simulink model "Intake"  (R2021a)
settings: Solver=FixedStepAuto  StartTime=0.0  StopTime=sim_time/4  FixedStep=stepsize  RelTol=1e-3
values from neighbouring files (symbols this model uses):
  AFR = 14.7    [Combustion_Engine.m]    (also in Combustion_Engine_V3.m)
  Bore = 82.7*10^-3    (= 0.0827)    [Combustion_Engine.m]    (also in Combustion_Engine_V3.m)
  Cd = 0.35    [Combustion_Engine.m]    (also in Combustion_Engine_V3.m)
  ConRod = 140*10^-3    (= 0.14)    [Combustion_Engine.m]    (also in Combustion_Engine_V3.m)
  CR = 10    [Combustion_Engine.m]    (also in Combustion_Engine_V3.m)
  CrankRadius = Stroke/2    (= 0.0465)    [Combustion_Engine.m]    (also in Combustion_Engine_V3.m)
  engine_speed = 3000    [Combustion_Engine.m]    (also in Combustion_Engine_V3.m)
  gma = 1.35    [Combustion_Engine.m]    (also in Combustion_Engine_V3.m)
  LHV = 44400*10^3    (= 44400000)    [Combustion_Engine.m]    (also in Combustion_Engine_V3.m)
  m_0 = P_0*(V_comp)/(R*T_air)    (= 5.9876570894e-05)    [Combustion_Engine.m]    (also in Combustion_Engine_V3.m)
  MAP = 80000    [Combustion_Engine.m]    (also in Combustion_Engine_V3.m)
  R = 287    [Combustion_Engine.m]    (also in Combustion_Engine_V3.m)
  Rho = 1.27    [Combustion_Engine.m]    (also in Combustion_Engine_V3.m)
  Stroke = 93*10^-3    (= 0.093)    [Combustion_Engine.m]    (also in Combustion_Engine_V3.m)
  T_air = 323    [Combustion_Engine.m]    (also in Combustion_Engine_V3.m)
  V2 = V_comp    (= 5.55061799844e-05)    [Combustion_Engine.m]    (also in Combustion_Engine_V3.m)
  V_comp = V_cyl/(CR-1)    (= 5.55061799844e-05)    [Combustion_Engine.m]    (also in Combustion_Engine_V3.m)
  V_cyl = (Bore/2)^2*pi*Stroke    (= 0.00049955561986)    [Combustion_Engine.m]    (also in Combustion_Engine_V3.m)
  Valve_dia = 30*10^-3    (= 0.03)    [Combustion_Engine.m]    (also in Combustion_Engine_V3.m)
  Valve_lift = 9*10^-3    (= 0.009)    [Combustion_Engine.m]    (also in Combustion_Engine_V3.m)
settings Model: Creator=rafik  LastModifiedBy=rafik
settings SolverCC: AlgebraicLoopSolver=TrustRegion
settings DataIOCC: ReturnWorkspaceOutputs=off
settings DebuggingCC: MaxConsecutiveZCsMsg=none

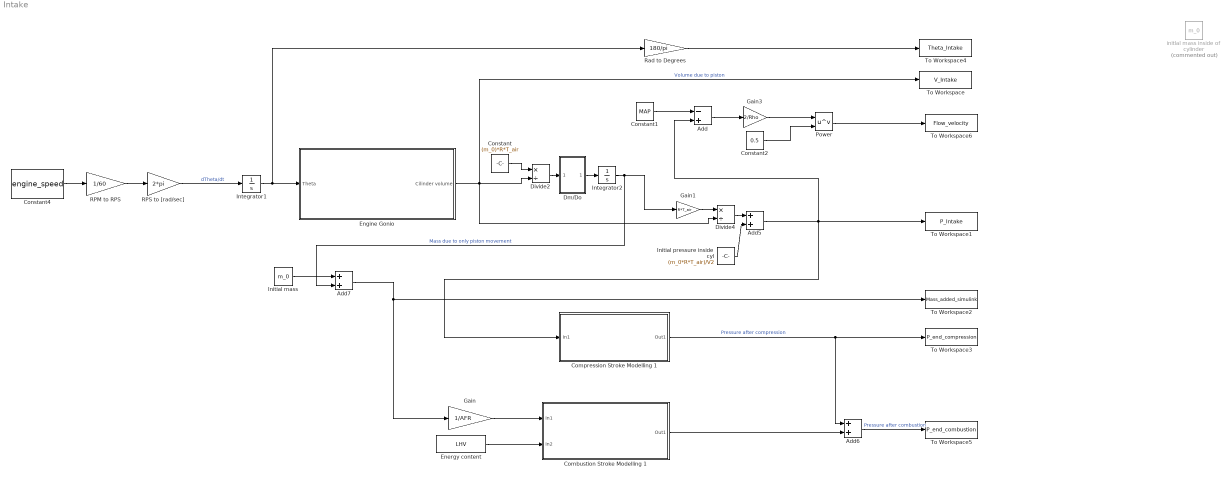
== system Intake ==
  Add : Sum  Inputs=-+
  Add5 : Sum
  Add6 : Sum
  Add7 : Sum
  Combustion Stroke Modelling 1 : Subsystem
  Compression Stroke Modelling 1 : Subsystem
  Constant : Constant  Value=(m_0)*R*T_air
  Constant1 : Constant  Value=MAP
  Constant2 : Constant  Value=0.5
  Constant4 : Constant  Value=engine_speed
  Divide2 : Product  Inputs=*/
  Divide4 : Product  Inputs=*/
  Dm/Do : Subsystem
  Energy content : Constant  Value=LHV
  Engine Gonio : Subsystem
  Gain : Gain  Gain=1/AFR
  Gain1 : Gain  Gain=R*T_air
  Gain3 : Gain  Gain=2/Rho
  "Initial mass " : Constant  Value=m_0
  Initial pressure inside cyl : Constant  Value=(m_0*R*T_air)/V2
  Integrator1 : Integrator  LimitOutput=on  UpperSaturationLimit=pi  LowerSaturationLimit=0
  Integrator2 : Integrator  LimitOutput=on  UpperSaturationLimit=1  LowerSaturationLimit=0
  Power : Math  Operator=pow  SaturateOnIntegerOverflow=on
  "RPM to RPS " : Gain  Gain=1/60
  RPS to [rad/sec] : Gain  Gain=2*pi
  "Rad to Degrees " : Gain  Gain=180/pi
  To Workspace : ToWorkspace  VariableName=V_Intake  SampleTime=-1
  To Workspace1 : ToWorkspace  VariableName=P_Intake  SampleTime=-1
  To Workspace2 : ToWorkspace  VariableName=Mass_added_simulink  SampleTime=-1
  To Workspace3 : ToWorkspace  VariableName=P_end_compression  SampleTime=-1
  To Workspace4 : ToWorkspace  VariableName=Theta_Intake  SampleTime=-1
  To Workspace5 : ToWorkspace  VariableName=P_end_combustion  SampleTime=-1
  To Workspace6 : ToWorkspace  VariableName=Flow_velocity  SampleTime=-1
  initlal mass inside of cylinder : Constant  Commented=on  Value=m_0
  wires:
  Energy content/1 -> Combustion Stroke Modelling 1/2(In2)
  Integrator1/1 -> "Rad to Degrees "/1, Engine Gonio/1(Theta)
  Constant4/1 -> "RPM to RPS "/1
  "RPM to RPS "/1 -> RPS to [rad/sec]/1
  RPS to [rad/sec]/1 -> Integrator1/1  "dTheta/dt"
  Constant/1 -> Divide2/1
  Engine Gonio/1(Cilinder volume) -> To Workspace/1, Divide2/2, Divide4/2  "Volume due to piston"
  Divide2/1 -> Dm/Do/1(In1)
  Gain1/1 -> Divide4/1
  Divide4/1 -> Add5/1
  Add5/1 -> Compression Stroke Modelling 1/1(In1), To Workspace1/1, Add/2
  Initial pressure inside cyl/1 -> Add5/2
  Compression Stroke Modelling 1/1(Out1) -> To Workspace3/1, Add6/1  "Pressure after compression"
  Integrator2/1 -> Add7/2, Gain1/1  "Mass due to only piston movement"
  Combustion Stroke Modelling 1/1(Out1) -> Add6/2
  Add6/1 -> To Workspace5/1  "Pressure after combustion"
  Gain/1 -> Combustion Stroke Modelling 1/1(In1)
  "Initial mass "/1 -> Add7/1
  Add7/1 -> Gain/1, To Workspace2/1
  "Rad to Degrees "/1 -> To Workspace4/1
  Dm/Do/1(Out1) -> Integrator2/1
  Constant1/1 -> Add/1
  Add/1 -> Gain3/1
  Gain3/1 -> Power/1
  Constant2/1 -> Power/2
  Power/1 -> To Workspace6/1

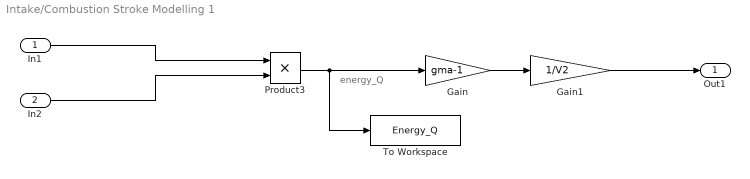
== system Intake/Combustion Stroke Modelling 1 ==
  note: energy_Q
  In1 : Inport
  In2 : Inport  Port=2
  Gain : Gain  Gain=gma-1
  Gain1 : Gain  Gain=1/V2
  Product3 : Product
  To Workspace : ToWorkspace  VariableName=Energy_Q  SaveFormat=Timeseries  SampleTime=-1
  Out1 : Outport
  wires:
  In2/1 -> Product3/2
  Product3/1 -> To Workspace/1, Gain/1
  In1/1 -> Product3/1
  Gain/1 -> Gain1/1
  Gain1/1 -> Out1/1

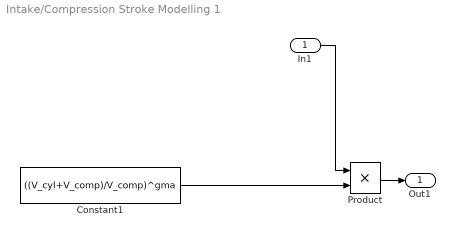
== system Intake/Compression Stroke Modelling 1 ==
  In1 : Inport
  Constant1 : Constant  Value=((V_cyl+V_comp)/V_comp)^gma
  Product : Product
  Out1 : Outport
  wires:
  Constant1/1 -> Product/2
  In1/1 -> Product/1
  Product/1 -> Out1/1

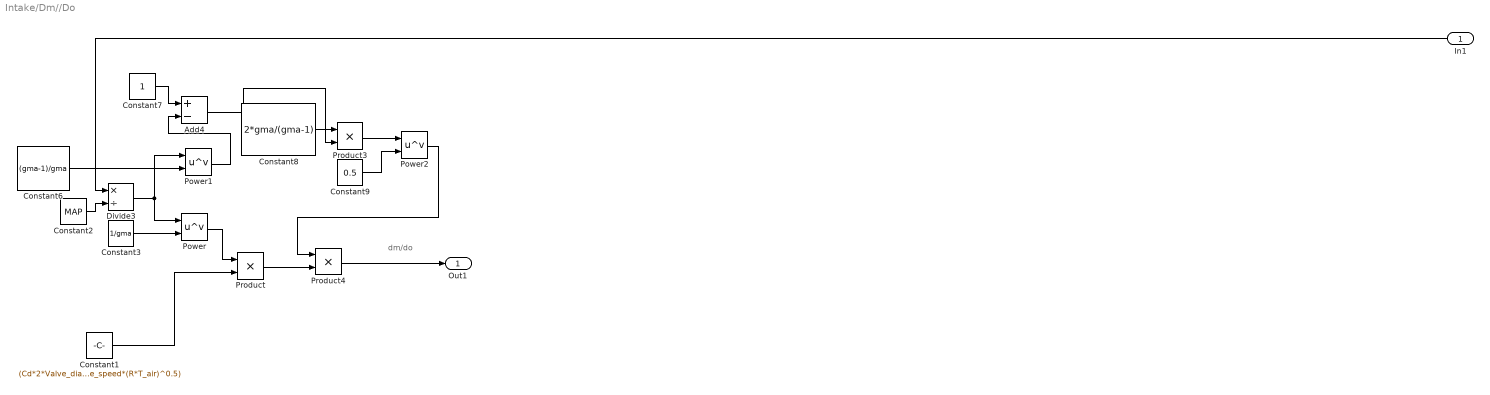
== system Intake/Dm//Do ==
  note: dm/do
  In1 : Inport
  Add4 : Sum  Inputs=+-
  Constant1 : Constant  Value=(Cd*2*Valve_dia*pi*Valve_lift*MAP)/(6*engine_speed*(R*T_air)^0.5)
  Constant2 : Constant  Value=MAP
  Constant3 : Constant  Value=1/gma
  Constant6 : Constant  Value=(gma-1)/gma
  Constant7 : Constant
  Constant8 : Constant  Value=2*gma/(gma-1)
  Constant9 : Constant  Value=0.5
  Divide3 : Product  Inputs=*/
  Power : Math  Operator=pow  SaturateOnIntegerOverflow=on
  Power1 : Math  Operator=pow  SaturateOnIntegerOverflow=on
  Power2 : Math  Operator=pow  SaturateOnIntegerOverflow=on
  Product : Product
  Product3 : Product
  Product4 : Product
  Out1 : Outport
  wires:
  Constant1/1 -> Product/2
  Power1/1 -> Add4/2
  Product/1 -> Product4/2
  Add4/1 -> Product3/2
  Constant8/1 -> Product3/1
  Divide3/1 -> Power1/1, Power/1
  Product3/1 -> Power2/1
  Constant9/1 -> Power2/2
  Power2/1 -> Product4/1
  Power/1 -> Product/1
  Constant3/1 -> Power/2
  Constant6/1 -> Power1/2
  Constant2/1 -> Divide3/2
  Constant7/1 -> Add4/1
  In1/1 -> Divide3/1
  Product4/1 -> Out1/1

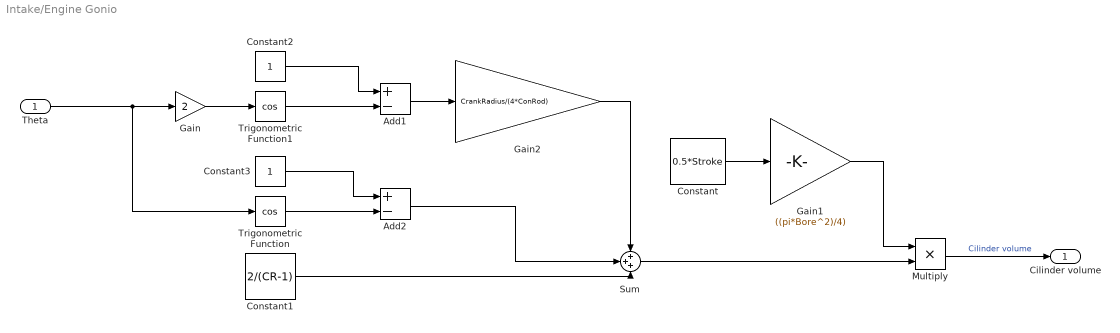
== system Intake/Engine Gonio ==
  Theta : Inport
  Add1 : Sum  Inputs=+-
  Add2 : Sum  Inputs=+-
  Constant : Constant  Value=0.5*Stroke
  Constant1 : Constant  Value=2/(CR-1)
  Constant2 : Constant
  Constant3 : Constant
  Gain : Gain  Gain=2
  Gain1 : Gain  Gain=((pi*Bore^2)/4)
  Gain2 : Gain  Gain=CrankRadius/(4*ConRod)
  Multiply : Product
  Sum : Sum  Inputs=+++
  Trigonometric Function : Trigonometry  Operator=cos
  Trigonometric Function1 : Trigonometry  Operator=cos
  Cilinder volume : Outport
  wires:
  Constant3/1 -> Add2/1
  Trigonometric Function/1 -> Add2/2
  Trigonometric Function1/1 -> Add1/2
  Multiply/1 -> Cilinder volume/1  "Cilinder volume"
  Sum/1 -> Multiply/2
  Constant2/1 -> Add1/1
  Gain2/1 -> Sum/1
  Add2/1 -> Sum/2
  Constant1/1 -> Sum/3
  Add1/1 -> Gain2/1
  Gain1/1 -> Multiply/1
  Gain/1 -> Trigonometric Function1/1
  Constant/1 -> Gain1/1
  Theta/1 -> Trigonometric Function/1, Gain/1
